simulink model "LorenzCircuitSim"  (R2014b)
settings: Solver=ode45  StartTime=0.0  StopTime=1000  RelTol=1e-12
values from neighbouring files (symbols this model uses):
  beta = 25.6    [RUN_021317.m]    (also in RUN_021417.m; RUN_022117.m)
  rho = 2    [RUN_021317.m]    (also in RUN_021417.m; RUN_022117.m)
  sig = 10    [RUN_021317.m]    (also in RUN_021417.m; RUN_022117.m)
  x0 = [.1,.2,.3]    [RUN_021317.m]    (also in RUN_021417.m; RUN_022117.m)
undefined symbols (not defined in the file or in its folder): betaResistor, rhoResistor, sigResistor
libraries: simulink x1
settings Model: Creator=Dan  LastModifiedBy=Dan

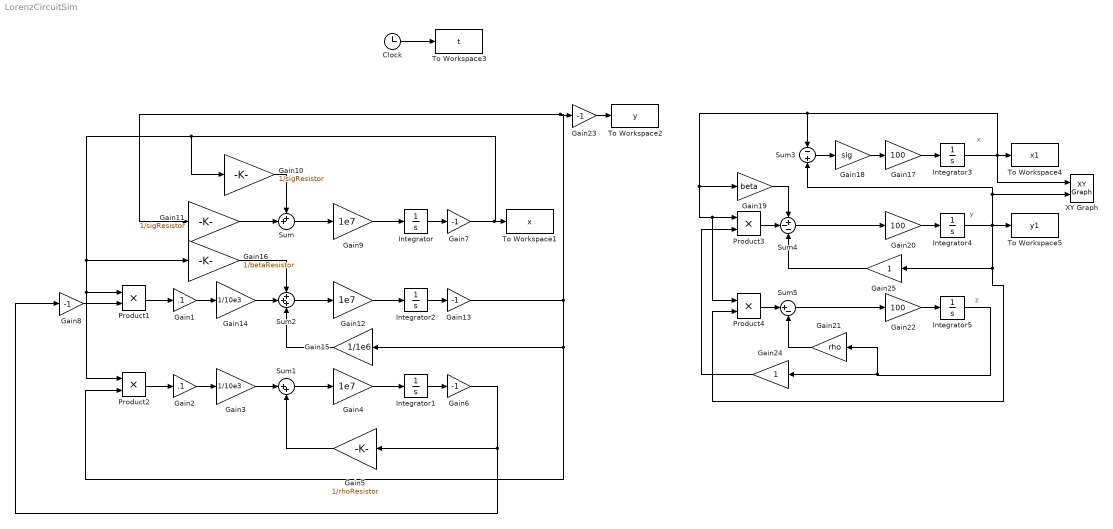
== system LorenzCircuitSim ==
  note: z
  note: y
  note: x
  Clock : Clock
  Gain1 : Gain  Gain=.1
  Gain10 : Gain  Gain=1/sigResistor
  Gain11 : Gain  Gain=1/sigResistor
  Gain12 : Gain  Gain=1e7
  Gain{6..8,13,23} (5 alike) : Gain  Gain=-1
  Gain14 : Gain  Gain=1/10e3
  Gain15 : Gain  Gain=1/1e6
  Gain16 : Gain  Gain=1/betaResistor
  Gain17 : Gain  Gain=100
  Gain18 : Gain  Gain=sig
  Gain19 : Gain  Gain=beta
  Gain2 : Gain  Gain=.1
  Gain20 : Gain  Gain=100
  Gain21 : Gain  Gain=rho
  Gain22 : Gain  Gain=100
  Gain24 : Gain
  Gain25 : Gain
  Gain3 : Gain  Gain=1/10e3
  Gain4 : Gain  Gain=1e7
  Gain5 : Gain  Gain=1/rhoResistor
  Gain9 : Gain  Gain=1e7
  Integrator : Integrator  InitialCondition=x0(1)
  Integrator1 : Integrator  InitialCondition=x0(3)
  Integrator2 : Integrator  InitialCondition=x0(2)
  Integrator3 : Integrator  InitialCondition=x0(1)
  Integrator4 : Integrator  InitialCondition=x0(2)
  Integrator5 : Integrator  InitialCondition=x0(3)
  Product{1..4} (4 alike) : Product
  Sum : Sum  Inputs=++|
  Sum1 : Sum  Inputs=|++
  Sum2 : Sum  Inputs=+++
  Sum3 : Sum  Inputs=-|+
  Sum4 : Sum  Inputs=+--
  Sum5 : Sum  Inputs=|+-
  To Workspace1 : ToWorkspace  VariableName=x  SampleTime=-1
  To Workspace2 : ToWorkspace  VariableName=y  SampleTime=-1
  To Workspace3 : ToWorkspace  VariableName=t  SampleTime=-1
  To Workspace4 : ToWorkspace  VariableName=x1  SampleTime=-1
  To Workspace5 : ToWorkspace  VariableName=y1  SampleTime=-1
  XY Graph : simulink/Sinks/XY Graph  xmin=-40  xmax=40  ymin=-40  ymax=40  st=-1
  wires:
  Product1/1 -> Gain1/1
  Product2/1 -> Gain2/1
  Gain2/1 -> Gain3/1
  Gain3/1 -> Sum1/1
  Sum1/1 -> Gain4/1
  Gain4/1 -> Integrator1/1
  Gain5/1 -> Sum1/2
  Integrator1/1 -> Gain6/1
  Integrator/1 -> Gain7/1
  Gain7/1 -> To Workspace1/1, Gain10/1, Gain16/1, Product2/1, Product1/1
  Gain8/1 -> Product1/2
  Gain6/1 -> Gain8/1, Gain5/1
  Gain9/1 -> Integrator/1
  Sum/1 -> Gain9/1
  Gain10/1 -> Sum/1
  Gain11/1 -> Sum/2
  Integrator2/1 -> Gain13/1
  Gain12/1 -> Integrator2/1
  Sum2/1 -> Gain12/1
  Gain14/1 -> Sum2/2
  Gain1/1 -> Gain14/1
  Gain15/1 -> Sum2/3
  Gain16/1 -> Sum2/1
  Gain13/1 -> Product2/2, Gain15/1, Gain23/1, Gain11/1
  Clock/1 -> To Workspace3/1
  Gain17/1 -> Integrator3/1
  Sum3/1 -> Gain18/1
  Gain18/1 -> Gain17/1
  Product3/1 -> Sum4/2
  Gain19/1 -> Sum4/1
  Sum4/1 -> Gain20/1
  Gain20/1 -> Integrator4/1
  Integrator5/1 -> Gain21/1, Gain24/1
  Integrator3/1 -> XY Graph/1, To Workspace4/1, Sum3/1, Gain19/1, Product3/1, Product4/1
  Product4/1 -> Sum5/1
  Gain21/1 -> Sum5/2
  Gain22/1 -> Integrator5/1
  Sum5/1 -> Gain22/1
  Integrator4/1 -> To Workspace5/1, Gain25/1, Product4/2, XY Graph/2, Sum3/2
  Gain23/1 -> To Workspace2/1
  Gain24/1 -> Product3/2
  Gain25/1 -> Sum4/3
